simulink model "diff_X"  (R2022b)
settings: Solver=VariableStepAuto  StartTime=0.0  StopTime=2  RelTol=1e-3
settings Model: Creator=Brigosha_Guest  LastModifiedBy=Brigosha_Guest

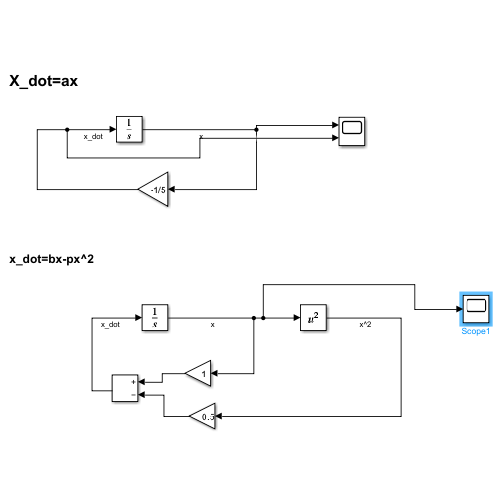
[thumbnail: Simulink's stored preview of the top-level diagram]
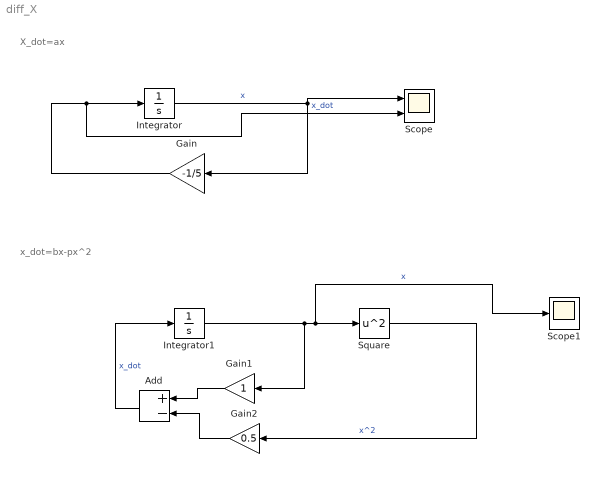
== system diff_X ==
  note: x_dot=bx-px^2
  note: X_dot=ax
  Add : Sum  Inputs=+-
  Gain : Gain  Gain=-1/5
  Gain1 : Gain
  Gain2 : Gain  Gain=0.5
  Integrator : Integrator  InitialCondition=1
  Integrator1 : Integrator  InitialCondition=100
  Scope : Scope  NumInputPorts=2
  Scope1 : Scope
  Square : Math  Operator=square
  wires:
  Gain/1 -> Scope/2, Integrator/1  "x_dot"
  Integrator/1 -> Gain/1, Scope/1  "x"
  Add/1 -> Integrator1/1  "x_dot"
  Integrator1/1 -> Gain1/1, Scope1/1, Square/1  "x"
  Square/1 -> Gain2/1  "x^2"
  Gain1/1 -> Add/1
  Gain2/1 -> Add/2
